simulink model "Controller_Model"  (R2025b)
settings: Solver=VariableStepAuto  StartTime=0.0  StopTime=10.0  RelTol=1e-3
undefined symbols (not defined in the file or in its folder): ISCS_Ad, ISCS_Bd, ISCS_Dd, ISCS_Tu, ISCS_Ty, Ts
settings Model: Creator=rapha  LastModifiedBy=rapha

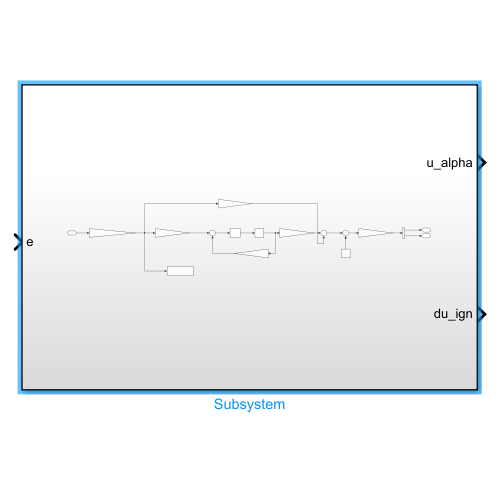
[thumbnail: Simulink's stored preview of the top-level diagram]
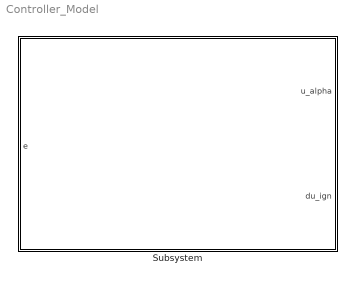
== system Controller_Model ==
  Subsystem : Subsystem

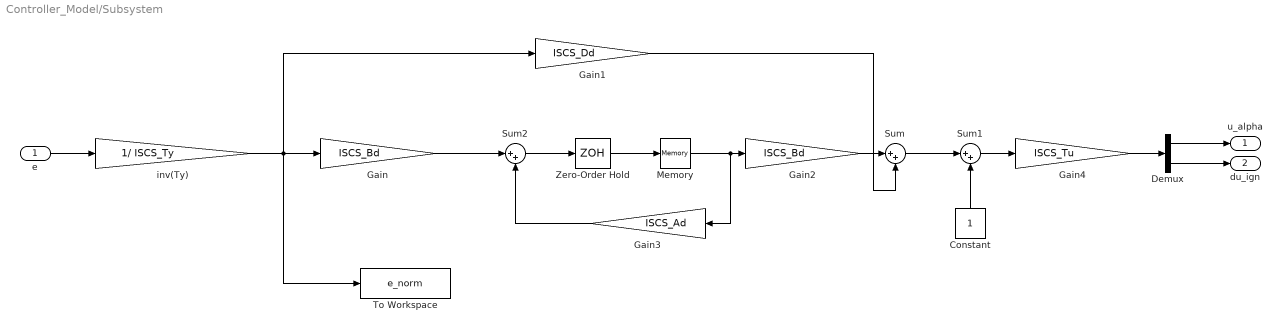
== system Controller_Model/Subsystem ==
  e : Inport
  Constant : Constant
  Demux : Demux  Outputs=2
  Gain : Gain  Gain=ISCS_Bd
  Gain1 : Gain  Gain=ISCS_Dd
  Gain2 : Gain  Gain=ISCS_Bd
  Gain3 : Gain  Gain=ISCS_Ad
  Gain4 : Gain  Gain=ISCS_Tu
  Memory : Memory
  Sum : Sum  Inputs=|++
  Sum1 : Sum  Inputs=|++
  Sum2 : Sum  Inputs=|++
  To Workspace : ToWorkspace  VariableName=e_norm  SaveFormat=Timeseries  SampleTime=-1
  Zero-Order Hold : ZeroOrderHold  SampleTime=Ts
  inv(Ty) : Gain  Gain=1/ ISCS_Ty
  u_alpha : Outport
  du_ign : Outport  Port=2
  wires:
  e/1 -> inv(Ty)/1
  inv(Ty)/1 -> To Workspace/1, Gain/1, Gain1/1
  Demux/1 -> u_alpha/1
  Demux/2 -> du_ign/1
  Zero-Order Hold/1 -> Memory/1
  Memory/1 -> Gain3/1, Gain2/1
  Constant/1 -> Sum1/2
  Sum1/1 -> Gain4/1
  Gain2/1 -> Sum/1
  Gain1/1 -> Sum/2
  Sum/1 -> Sum1/1
  Gain3/1 -> Sum2/2
  Gain/1 -> Sum2/1
  Sum2/1 -> Zero-Order Hold/1
  Gain4/1 -> Demux/1
